simulink model "Senorless"  (R2023a)
settings: Solver=FixedStepDiscrete  StartTime=0.0  StopTime=2  FixedStep=1/FOC_FRQ  RelTol=1e-3
values from neighbouring files (symbols this model uses):
  ADC_REF = 3.6    [Senorless.sldd]
  ADC_SAMPLE_MAX = 32767.0    [Senorless.sldd]
  AMP_GAIN = 32.0    [Senorless.sldd]
  CURR_INPUT = 3276.0    [Senorless.sldd]
  CURR_KI = 380.0    [Senorless.sldd]
  CURR_KP = 0.04    [Senorless.sldd]
  CURR_LIMIT = 1.1    [Senorless.sldd]
  CURR_OVER = 34.0    [Senorless.sldd]
  CURR_POINT_GAIN = 7.0    [Senorless.sldd]
  CURR_STEP = 32760.0    [Senorless.sldd]
  CURR_UNDER = 0.03    [Senorless.sldd]
  CURR_WIDTH = 250.0    [Senorless.sldd]
  FOC_FRQ = 36000.0    [Senorless.sldd]
  GAMMA = 32767.0    [Senorless.sldd]
  HFI_ID = 2.125    [Senorless.sldd]
  IMAX = 34.0    [Senorless.sldd]
  LPF_FRQ = 300.0    [Senorless.sldd]
  MOTOR_DAMPER = 8.3E-7    [Senorless.sldd]
  MOTOR_FLUX = 0.0012713112    [Senorless.sldd]
  MOTOR_INERTIA = 1.02E-6    [Senorless.sldd]
  MOTOR_LS = 1.8E-5    [Senorless.sldd]
  MOTOR_PN = 7.0    [Senorless.sldd]
  MOTOR_RS = 0.065    [Senorless.sldd]
  NS_COMP_UD = 0.531    [Senorless.sldd]
  PLL_LIMIT = 0.95    [Senorless.sldd]
  PLL_WIDTH = 500.0    [Senorless.sldd]
  PWM_FRQ = 96000000.0    [Senorless.sldd]
  RS_HUNT = 0.002    [Senorless.sldd]
  SMOK_FRQ = 1200.0    [Senorless.sldd]
  SPD_LIMIT = 0.8    [Senorless.sldd]
  SPD_LPF_LEVEL = 15.0    [Senorless.sldd]
  SPD_MAX = 8100.0    [Senorless.sldd]
  SPD_MIN = -8100.0    [Senorless.sldd]
  SPD_REDUCE = 380.0    [Senorless.sldd]
  SPD_STEP = 3.0    [Senorless.sldd]
  SPD_WIDTH = 10.0    [Senorless.sldd]
  TS_POINT_GAIN = 10.0    [Senorless.sldd]
  UDC = 17.0    [Senorless.sldd]
  UDC_GAIN = 21.0    [Senorless.sldd]
  UDC_POINT_GAIN = 10.0    [Senorless.sldd]
undefined symbols (not defined in the file or in its folder): curr_q_ki, curr_q_kp, DiscIntNeverNeededParam, magnitude, PLL_LPF_LEVEL, Udc
libraries: simulink x20, slpidlib x5, mcbcontrolslib x4, mcbplantlib x1, autolibpmsminterior x1, autolibpmsmexterior x1, spspowerguiLib x1
(part 4 of 7)

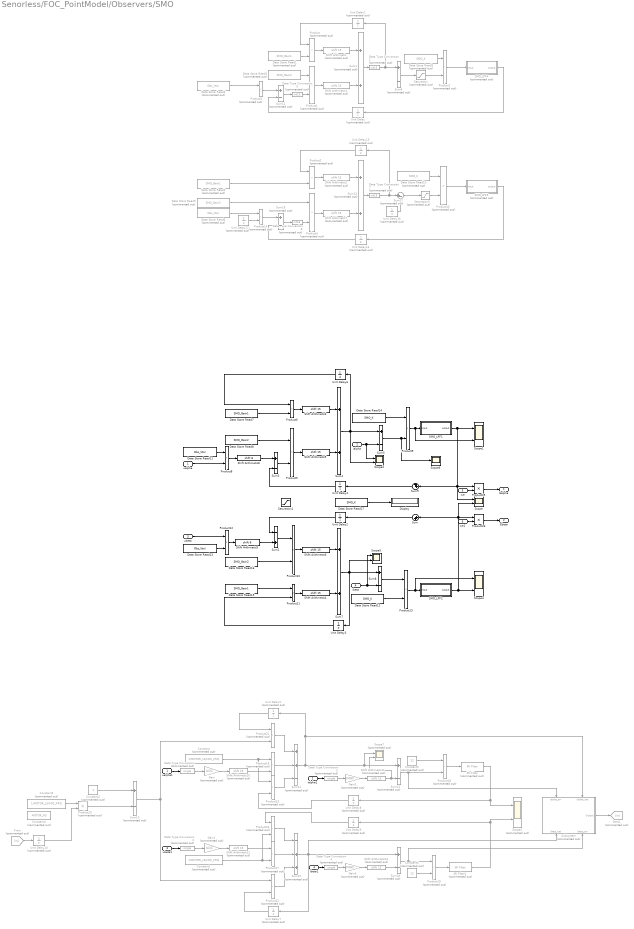
== system Senorless/FOC_PointModel/Observers/SMO ==
  ualpha : Inport
  ialpha : Inport  Port=2
  ubeta : Inport  Port=3
  ibeta : Inport  Port=4
  we : Inport  Port=5
  Constant : Constant  Commented=on  Value=1/MOTOR_LS/FOC_FRQ
  Constant1 : Constant  Commented=on  Value=1/MOTOR_LS/FOC_FRQ
  Constant2 : Constant  Commented=on  OutDataTypeStr=single
  Constant3 : Constant  Commented=on  Value=1/MOTOR_LS/FOC_FRQ
  Constant4 : Constant  Commented=on  Value=MOTOR_RS
  Constant5 : Constant  Commented=on  Value=12  OutDataTypeStr=single
  Constant6 : Constant  Commented=on  Value=12  OutDataTypeStr=single
  Data Store Read1 : DataStoreRead  Commented=on  DataStoreName=SMO_Gain1  IndexOptions=Index vector (dialog)  Indices=1  OutputSizes=1
  Data Store Read10 : DataStoreRead  Commented=on  DataStoreName=SMO_K  IndexOptions=Index vector (dialog)  Indices=1  OutputSizes=1
  Data Store Read11 : DataStoreRead  DataStoreName=Obs_VtoI  IndexOptions=Index vector (dialog)  Indices=1  OutputSizes=1
  Data Store Read12 : DataStoreRead  DataStoreName=SMO_K  IndexOptions=Index vector (dialog)  Indices=1  OutputSizes=1
  Data Store Read13 : DataStoreRead  DataStoreName=Obs_VtoI  IndexOptions=Index vector (dialog)  Indices=1  OutputSizes=1
  Data Store Read14 : DataStoreRead  DataStoreName=SMO_K  IndexOptions=Index vector (dialog)  Indices=1  OutputSizes=1
  Data Store Read15 : DataStoreRead  DataStoreName=SMO_Gain1  IndexOptions=Index vector (dialog)  Indices=1  OutputSizes=1
  Data Store Read16 : DataStoreRead  DataStoreName=SMO_Gain2  IndexOptions=Index vector (dialog)  Indices=1  OutputSizes=1
  Data Store Read17 : DataStoreRead  DataStoreName=SMO_K  IndexOptions=Index vector (dialog)  Indices=1  OutputSizes=1
  Data Store Read2 : DataStoreRead  Commented=on  DataStoreName=SMO_Gain1  IndexOptions=Index vector (dialog)  Indices=1  OutputSizes=1
  Data Store Read3 : DataStoreRead  Commented=on  DataStoreName=SMO_Gain2  IndexOptions=Index vector (dialog)  Indices=1  OutputSizes=1
  Data Store Read4 : DataStoreRead  Commented=on  DataStoreName=Obs_VtoI  IndexOptions=Index vector (dialog)  Indices=1  OutputSizes=1
  Data Store Read5 : DataStoreRead  Commented=on  DataStoreName=SMO_Gain2  IndexOptions=Index vector (dialog)  Indices=1  OutputSizes=1
  Data Store Read6 : DataStoreRead  Commented=on  DataStoreName=Obs_VtoI  IndexOptions=Index vector (dialog)  Indices=1  OutputSizes=1
  Data Store Read7 : DataStoreRead  DataStoreName=SMO_Gain1  IndexOptions=Index vector (dialog)  Indices=1  OutputSizes=1
  Data Store Read8 : DataStoreRead  DataStoreName=SMO_Gain2  IndexOptions=Index vector (dialog)  Indices=1  OutputSizes=1
  Data Store Read9 : DataStoreRead  Commented=on  DataStoreName=SMO_K  IndexOptions=Index vector (dialog)  Indices=1  OutputSizes=1
  Data Type Conversion{,2..4} (4 alike) : DataTypeConversion  Commented=on  OutDataTypeStr=single  SaturateOnIntegerOverflow=off  RndMeth=Floor
  Data Type Conversion{1,5,7..8} (4 alike) : DataTypeConversion  Commented=on  OutDataTypeStr=int16  SaturateOnIntegerOverflow=off
  Display : Display
  From : From  Commented=on  GotoTag=rs
  Gain : Gain  Commented=on  Gain=UDC
  Gain1 : Gain  Commented=on  Gain=UDC
  Gain2 : Gain  Commented=on  Gain=IMAX
  Gain3 : Gain  Commented=on  Gain=IMAX
  Goto1 : Goto  Commented=on  GotoTag=rs
  IIR Filter : mcbcontrolslib/IIR Filter  Commented=on  VariantControl=Low Pass Filter  VariantSelect=Low-pass  Filter_constant=0.07  advancedSettings=off  Ts=50e-6  cutOff_freq=239.5881
      settings: LibrarySourceBlock=mcbhdllib/Signal Management/IIR Filter
  IIR Filter1 : mcbcontrolslib/IIR Filter  Commented=on  VariantControl=Low Pass Filter  VariantSelect=Low-pass  Filter_constant=0.07  advancedSettings=off  Ts=50e-6  cutOff_freq=239.5881
      settings: LibrarySourceBlock=mcbhdllib/Signal Management/IIR Filter
  Product{,1..4,7,14..15} (8 alike) : Product  Commented=on  OutDataTypeStr=int32  RndMeth=Zero
  Product{5..6,8..13,25..26} (10 alike) : Product  OutDataTypeStr=int32  RndMeth=Zero
  Product{16..24} (9 alike) : Product  Commented=on
  SMO_LPF1 : Subsystem
  SMO_LPF2 : Subsystem
  SMO_LPF4 : Subsystem  Commented=on  TreatAsAtomicUnit=on
  SMO_LPF5 : Subsystem  Commented=on  TreatAsAtomicUnit=on
  Saturation : Saturate  Commented=on  UpperLimit=32768*0.5  LowerLimit=-32768*0.5  OutDataTypeStr=int16  RndMeth=Zero
  Saturation1 : Saturate  UpperLimit=32767  LowerLimit=-32767  OutDataTypeStr=int32  RndMeth=Zero
  Saturation3 : Saturate  Commented=on  UpperLimit=32768*0.5  LowerLimit=-32768*0.5  OutDataTypeStr=int16  RndMeth=Zero
  Scope{,1..2,4..5} (5 alike) : Scope  NumInputPorts=2
  Scope3 : Scope  Commented=on  NumInputPorts=2
  Scope6 : Scope
  Scope7 : Scope  Commented=on  NumInputPorts=2
  Shift Arithmetic{,1..2,7,10..13} (8 alike) : ArithShift  Commented=on  BitShiftNumber=15
  Shift Arithmetic{3..6} (4 alike) : ArithShift  BitShiftNumber=15  DiagnosticForOORShift=Error
  Shift Arithmetic8 : ArithShift  BitShiftNumber=8
  Shift Arithmetic9 : ArithShift  BitShiftNumber=8
  Subsystem : Subsystem  Commented=on
      settings: PortSchema="{\"entries\":[{\"content\":{\"sides\":[{\"content\":{},\"type\":\"ConnectorPlacement.EquallySpacedRectSide\",\"uuid\":\"b8d9eb56-9873-4626-b110-f5e82f41559d\"},{\"content\":{\"connectorIds\":[\"Out1\"],\"side\":\"RIGHT\"},\"type\":\"ConnectorPlacement.EquallySpacedRectSide\",\"uuid\":\"658789fc-224b-44e9-b365-546b63f28a3f\"},{\"content\":{\"connectorIds\":[\"In1\",\"In2\"],\"side\":\"TOP\"},\"type\":\"ConnectorPlacement.EquallySpacedRectSide\",\"uuid\":\"05c41f48-0bd2-48b6-962d-dae447ff7d68\"},{\"content\":{\"connectorIds\":[\"In3\",\"In4\"],\"side\":\"BOTTOM\"},\"type\":\"ConnectorPlacement.EquallySpacedRectSide\",\"uuid\":\"829c9f03-f344-43ec-9cb0-3f5e0857c861\"}]},\"type\":\"ConnectorPlacement.EquallySpacedConnector\",\"uuid\":\"ff8d46c8-3816-4d27-98d8-4daa626fea9c\"}],\"packageUris\":[\"http://schema.mathworks.com/mf0/Connector/R2020b\"],\"version\":\"1.0\"}"
  Sum : Sum  Inputs=|++
  Sum1 : Sum  Commented=on
  Sum10 : Sum  Commented=on  Inputs=+-
  Sum11 : Sum  Commented=on  Inputs=++-
  Sum12 : Sum  Commented=on  Inputs=+-
  Sum13 : Sum  Commented=on
  Sum14 : Sum  Commented=on  Inputs=+-  RndMeth=Zero
  Sum15 : Sum  Commented=on  Inputs=-++
  Sum16 : Sum  Commented=on  Inputs=+-
  Sum17 : Sum  Commented=on  Inputs=|+-  OutDataTypeStr=int16  RndMeth=Zero
  Sum18 : Sum  Commented=on  Inputs=+-  RndMeth=Zero
  Sum2 : Sum  Inputs=-+
  Sum3 : Sum  Inputs=+-  OutDataTypeStr=int32  RndMeth=Zero
  Sum4 : Sum  OutDataTypeStr=int32  RndMeth=Zero
  Sum5 : Sum  Inputs=+-  OutDataTypeStr=int32  RndMeth=Zero
  Sum6 : Sum  Commented=on  Inputs=+-  OutDataTypeStr=int16  RndMeth=Zero
  Sum7 : Sum  OutDataTypeStr=int32
  Sum8 : Sum  Inputs=+-  OutDataTypeStr=int32  RndMeth=Zero
  Sum9 : Sum  Inputs=++|
  Unit Delay{,1,5,7..9,14..17} (10 alike) : UnitDelay  Commented=on  SampleTime=-1  HasFrameUpgradeWarning=on
  Unit Delay10 : UnitDelay  Commented=on  InitialCondition=MOTOR_RS  SampleTime=-1  HasFrameUpgradeWarning=on
  Unit Delay{2..4,6} (4 alike) : UnitDelay  SampleTime=-1  HasFrameUpgradeWarning=on
  ialpha1 : InportShadow  Port=2
  ibeta1 : InportShadow  Port=4
  ualpha1 : InportShadow
  ubeta1 : InportShadow  Port=3
  we1 : InportShadow  Port=5
  Ealpha : Outport
  Ebeta : Outport  Port=2
  wires:
  Shift Arithmetic1/1 -> Sum1/2
  Shift Arithmetic2/1 -> Sum13/1
  Data Store Read1/1 -> Product/2
  Data Store Read4/1 -> Product3/1
  Product1/1 -> Shift Arithmetic1/1
  Product3/1 -> Sum12/1
  Unit Delay/1 -> Sum12/2
  Data Type Conversion1/1 -> Sum6/1, Unit Delay1/1
  Sum1/1 -> Data Type Conversion1/1
  Unit Delay1/1 -> Product/1
  Product/1 -> Shift Arithmetic/1
  Saturation3/1 -> Product15/2
  Data Type Conversion7/1 -> Unit Delay15/1, Sum17/1
  Data Store Read5/1 -> Product4/1
  Saturation/1 -> Product7/2
  Product2/1 -> Shift Arithmetic2/1
  Sum12/1 -> Data Type Conversion5/1
  Sum17/1 -> Saturation3/1
  Data Type Conversion5/1 -> Product1/2
  Unit Delay15/1 -> Product2/1
  Shift Arithmetic/1 -> Sum1/1
  Unit Delay14/1 -> Sum16/2
  Sum13/1 -> Data Type Conversion7/1
  Data Type Conversion8/1 -> Product4/2
  Data Store Read2/1 -> Product2/2
  Shift Arithmetic7/1 -> Sum13/2
  Product4/1 -> Shift Arithmetic7/1
  Unit Delay17/1 -> Product14/2
  Product14/1 -> Sum16/1
  Sum16/1 -> Data Type Conversion8/1
  Data Store Read6/1 -> Product14/1
  Unit Delay16/1 -> Sum17/2
  Data Store Read3/1 -> Product1/1
  Data Store Read9/1 -> Product7/1
  Data Store Read10/1 -> Product15/1
  Product15/1 -> SMO_LPF5/1(input)
  Product7/1 -> SMO_LPF4/1(input)
  SMO_LPF4/1(output) -> Unit Delay/1
  SMO_LPF5/1(output) -> Unit Delay14/1
  Data Store Read8/1 -> Product5/1
  Product6/1 -> Shift Arithmetic3/1
  Product5/1 -> Shift Arithmetic5/1
  Sum6/1 -> Saturation/1
  Product10/1 -> Shift Arithmetic6/1
  Product11/1 -> Shift Arithmetic4/1
  Shift Arithmetic3/1 -> Sum4/1
  Shift Arithmetic5/1 -> Sum4/2
  Data Store Read17/1 -> Display/1
  Data Store Read14/1 -> Product9/1
  Sum7/1 -> Scope5/2, Unit Delay3/1, Sum8/1
  Sum4/1 -> Sum5/1, Scope2/2, Unit Delay6/1
  Sum/1 -> Unit Delay2/1
  Sum9/1 -> Unit Delay4/1
  ialpha/1 -> Scope2/1, Sum5/2
  ibeta/1 -> Scope5/1, Sum8/2
  Unit Delay6/1 -> Product6/1
  Product13/1 -> SMO_LPF2/1(input), Scope4/1
  Shift Arithmetic6/1 -> Sum7/1
  Data Store Read16/1 -> Product10/2
  Shift Arithmetic4/1 -> Sum7/2
  Unit Delay3/1 -> Product11/2
  Data Store Read12/1 -> Product13/2
  Subsystem/1(Output) -> Goto1/1
  Data Store Read7/1 -> Product6/2
  Data Store Read15/1 -> Product11/1
  Sum8/1 -> Product13/1
  Sum3/1 -> Product5/2
  Product8/1 -> Shift Arithmetic8/1
  Data Store Read11/1 -> Product8/1
  Unit Delay4/1 -> Sum3/2
  Sum2/1 -> Product10/1
  Shift Arithmetic9/1 -> Sum2/2
  Product12/1 -> Shift Arithmetic9/1
  Data Store Read13/1 -> Product12/2
  Unit Delay2/1 -> Sum2/1
  SMO_LPF2/1(output) -> Scope4/2, Product26/1, Sum/1, Scope/2
  Sum5/1 -> Scope6/1, Product9/2
  ualpha1/1 -> Data Type Conversion/1
  ubeta1/1 -> Data Type Conversion2/1
  ialpha1/1 -> Data Type Conversion3/1
  ibeta1/1 -> Data Type Conversion4/1
  Gain/1 -> Shift Arithmetic10/1
  Gain1/1 -> Shift Arithmetic12/1
  Gain3/1 -> Shift Arithmetic13/1
  Gain2/1 -> Shift Arithmetic11/1
  Shift Arithmetic10/1 -> Product16/2
  Constant/1 -> Product23/1, Product16/1
  Constant1/1 -> Product24/2, Product17/2
  Constant2/1 -> Sum10/1
  Product20/1 -> Sum10/2
  Constant3/1 -> Product20/1
  Sum10/1 -> Product22/1, Product21/2
  Product16/1 -> Sum11/2
  Product21/1 -> Sum11/1
  Sum11/1 -> Scope7/1, Sum14/1, Subsystem/2(ialpha_hat), Unit Delay5/1
  Unit Delay5/1 -> Product21/1
  Shift Arithmetic11/1 -> Scope7/2, Sum14/2
  Constant5/1 -> Product18/1
  Product18/1 -> IIR Filter/1
  IIR Filter/1 -> Scope3/1, Unit Delay8/1
  Sum15/1 -> Subsystem/3(ibeta_hat), Unit Delay7/1, Sum18/1
  Shift Arithmetic13/1 -> Sum18/2
  Product17/1 -> Sum15/2
  Product22/1 -> Sum15/3
  Constant6/1 -> Product19/2
  Product19/1 -> IIR Filter1/1
  IIR Filter1/1 -> Scope3/2, Unit Delay9/1
  Unit Delay7/1 -> Product22/2
  Data Type Conversion/1 -> Gain/1
  Data Type Conversion2/1 -> Gain1/1
  Data Type Conversion3/1 -> Gain2/1
  Data Type Conversion4/1 -> Gain3/1
  Unit Delay8/1 -> Product23/2
  SMO_LPF1/1(output) -> Product25/1, Sum9/2, Scope/1, Scope1/1
  ubeta/1 -> Product12/1
  ualpha/1 -> Product8/2
  Product9/1 -> Scope1/2, SMO_LPF1/1(input)
  Shift Arithmetic8/1 -> Sum3/1
  Shift Arithmetic12/1 -> Product17/1
  Unit Delay9/1 -> Product24/1
  Product24/1 -> Sum15/1
  Product23/1 -> Sum11/3
  From/1 -> Unit Delay10/1
  Sum14/1 -> Product18/2, Subsystem/1(ialpha_err)
  Sum18/1 -> Product19/1, Subsystem/4(ibeta_err)
  Unit Delay10/1 -> Product20/2
  we/1 -> Product25/2
  Product25/1 -> Ealpha/1
  Product26/1 -> Ebeta/1
  we1/1 -> Product26/2

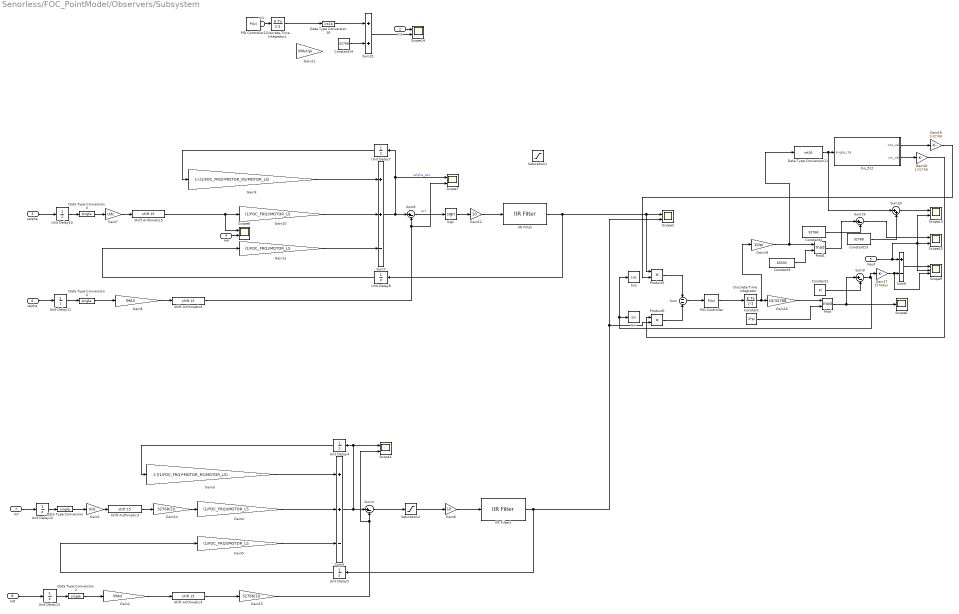
== system Senorless/FOC_PointModel/Observers/Subsystem ==
  In1 : Inport
  In2 : Inport  Port=2
  ualpha : Inport  Port=3
  In4 : Inport  Port=4
  Input : Inport  Port=5
  ialpha : Inport  Port=6
  In7 : Inport  Port=7
  In8 : Inport  Port=8
  Constant : Constant  Value=2*pi  OutDataTypeStr=single
  Constant1 : Constant  Value=pi  OutDataTypeStr=single
  Constant13 : Constant  Value=32768  OutDataTypeStr=int16
  Constant14 : Constant  Value=32768  OutDataTypeStr=int16
  Constant3 : Constant  Value=65535  OutDataTypeStr=single
  Constant4 : Constant  Value=32768
  Cos : Trigonometry  Operator=cos
  Data Type Conversion{,2..4} (4 alike) : DataTypeConversion  OutDataTypeStr=single  SaturateOnIntegerOverflow=off  RndMeth=Floor
  Data Type Conversion11 : DataTypeConversion  OutDataTypeStr=int16  SaturateOnIntegerOverflow=off  RndMeth=Floor
  Data Type Conversion16 : DataTypeConversion  OutDataTypeStr=int16  SaturateOnIntegerOverflow=off
  Discrete-Time Integrator : DiscreteIntegrator  SampleTime=-1  ICPrevOutput=DiscIntNeverNeededParam  ICPrevScaledInput=DiscIntNeverNeededParam
  Discrete-Time Integrator1 : DiscreteIntegrator  SampleTime=-1  OutDataTypeStr=int32  RndMeth=Zero  ICPrevOutput=DiscIntNeverNeededParam  ICPrevScaledInput=DiscIntNeverNeededParam
  Gain1 : Gain  Gain=Udc
  Gain10 : Gain  Gain=(1/FOC_FRQ)/MOTOR_LS
  Gain11 : Gain  Gain=(1/FOC_FRQ)/MOTOR_LS  OutDataTypeStr=single
  Gain12 : Gain  Gain=10
  Gain14 : Gain  Gain=32768/10
  Gain15 : Gain  Gain=32768/10
  Gain16 : Gain  Gain=10/32768
  Gain17 : Gain  Gain=32768/pi
  Gain18 : Gain  Gain=10/pi
  Gain19 : Gain  Gain=1/32768  OutDataTypeStr=single
  Gain2 : Gain  Gain=IMAX
  Gain20 : Gain  Gain=1/32768  OutDataTypeStr=single
  Gain21 : Gain  Gain=IMAX/pi  OutDataTypeStr=int32  RndMeth=Zero
  Gain3 : Gain  Gain=1-((1/FOC_FRQ)*MOTOR_RS/MOTOR_LS)  OutDataTypeStr=single
  Gain4 : Gain  Gain=(1/FOC_FRQ)/MOTOR_LS
  Gain5 : Gain  Gain=(1/FOC_FRQ)/MOTOR_LS  OutDataTypeStr=single
  Gain6 : Gain  Gain=10
  Gain7 : Gain  Gain=Udc
  Gain8 : Gain  Gain=IMAX
  Gain9 : Gain  Gain=1-((1/FOC_FRQ)*MOTOR_RS/MOTOR_LS)  OutDataTypeStr=single
  IIR Filter : mcbcontrolslib/IIR Filter  VariantControl=Low Pass Filter  VariantSelect=Low-pass  Filter_constant=0.1  advancedSettings=off  Ts=50e-6  cutOff_freq=353.6777
      settings: LibrarySourceBlock=mcbhdllib/Signal Management/IIR Filter
  IIR Filter1 : mcbcontrolslib/IIR Filter  VariantControl=Low Pass Filter  VariantSelect=Low-pass  Filter_constant=0.149  advancedSettings=off  Ts=50e-6  cutOff_freq=557.3228
      settings: LibrarySourceBlock=mcbhdllib/Signal Management/IIR Filter
  Mod : Math  Operator=mod
  Mod1 : Math  Operator=mod
  PID Controller : slpidlib/PID Controller  Controller=PI  Form=Parallel  TimeDomain=Discrete-time  UseExternalTs=off  SampleTime=-1  IntegratorMethod=Forward Euler  FilterMethod=Forward Euler  ControllerParametersSource=internal  P=2*0.707*100  I=100*100  UseKiTs=off  D=0  N=100  UseFilter=on  TunerSelectOption=Transfer Function Based (PID Tuner App)  InitialConditionSource=internal  InitialConditionForIntegrator=0  InitialConditionForFilter=0  DifferentiatorICPrevScaledInput=0  ExternalReset=none  TrackingMode=off  Kt=1  LimitOutput=off  SatLimitsSource=internal  UpperSaturationLimit=inf  LowerSaturationLimit=-inf  LinearizeAsGain=on  AntiWindupMode=none  Kb=1  LimitIntegrator=off  UpperIntegratorSaturationLimit=inf  LowerIntegratorSaturationLimit=-inf  POutMin=[]  POutMax=[]  IOutMin=[]  IOutMax=[]  DOutMin=[]  DOutMax=[]  NOutMin=[]  NOutMax=[]  SumOutMin=[]  SumOutMax=[]  SaturationOutMin=[]  SaturationOutMax=[]  PParamMin=[]  PParamMax=[]  IParamMin=[]  IParamMax=[]  DParamMin=[]  DParamMax=[]  NParamMin=[]  NParamMax=[]  KbParamMin=[]  KbParamMax=[]  KtParamMin=[]  KtParamMax=[]  KbOutMin=[]  KbOutMax=[]  KtOutMin=[]  KtOutMax=[]  IntegratorOutMin=[]  IntegratorOutMax=[]  FilterOutMin=[]  FilterOutMax=[]  SumI1OutMin=[]  SumI1OutMax=[]  SumI2OutMin=[]  SumI2OutMax=[]  SumI3OutMin=[]  SumI3OutMax=[]  SumI4OutMin=[]  SumI4OutMax=[]  SumDOutMin=[]  SumDOutMax=[]  DifferentiatorOutMin=[]  DifferentiatorOutMax=[]  FilterDiffOutCoefMin=[]  FilterDiffOutCoefMax=[]  ReciprocalOutMin=[]  ReciprocalOutMax=[]  SumDenOutMin=[]  SumDenOutMax=[]  SumNumOutMin=[]  SumNumOutMax=[]  DivideOutMin=[]  DivideOutMax=[]  UdiffTsProdOutMin=[]  UdiffTsProdOutMax=[]  NTsProdOutMin=[]  NTsProdOutMax=[]  UintegralTsProdOutMin=[]  UintegralTsProdOutMax=[]  UngainTsProdOutMin=[]  UngainTsProdOutMax=[]  ClampingZeroOutDataTypeStr=Inherit: Inherit via back propagation  ClampingZeroOutMin=[]  ClampingZeroOutMax=[]  FilterDenConstantOutDataTypeStr=Inherit: Inherit via back propagation  FilterDenConstantOutMin=[]  FilterDenConstantOutMax=[]  PCopyOutDataTypeStr=Inherit: Inherit via back propagation  PCopyOutMin=[]  PCopyOutMax=[]  NCopyOutDataTypeStr=Inherit: Inherit via back propagation  NCopyOutMin=[]  NCopyOutMax=[]  IntegratorContinuousStateAttributes=''  IntegratorStateMustResolveToSignalObject=off  IntegratorRTWStateStorageClass=Auto  FilterContinuousStateAttributes=''  FilterStateMustResolveToSignalObject=off  FilterRTWStateStorageClass=Auto  ParallelPVariant=InternalParameters  IdealPVariant=Disabled  IVariant=InternalParameters  DVariant=Disabled  IntegratorVariant=Discrete  SatVariant=Disabled  AWVariant=Passthrough  PCopyVariant=Disabled  TRVariant=Disabled  FdbkBlocksVariant=Forward  IdealPFdbkVariant=Disabled  SatFdbkVariant=Disabled  DerivativeFilterVariant=Disabled  NVariant=Disabled  NCopyVariant=Disabled_SignalSpec  FilterICVariant=Disabled  IntegratorICVariant=InternalICs  ExternalResetVariant=Disabled  TRSumVariant=Passthrough  SumFdbkVariant=Disabled  SumVariant=Sum_PI  TsampFilterVariant=InternalTs  TsampNgainVariant=Passthrough  TsampIntegralVariant=Disabled_SignalSpec  ExternalSaturationOutDataTypeStr=Inherit: Same as second input
  PID Controller1 : slpidlib/PID Controller  Controller=PI  Form=Parallel  TimeDomain=Discrete-time  UseExternalTs=off  SampleTime=-1  IntegratorMethod=Forward Euler  FilterMethod=Forward Euler  ControllerParametersSource=internal  P=2*0.707*100  I=100*100  UseKiTs=off  D=0  N=100  UseFilter=on  TunerSelectOption=Transfer Function Based (PID Tuner App)  InitialConditionSource=internal  InitialConditionForIntegrator=0  InitialConditionForFilter=0  DifferentiatorICPrevScaledInput=0  ExternalReset=none  TrackingMode=off  Kt=1  LimitOutput=off  SatLimitsSource=internal  UpperSaturationLimit=inf  LowerSaturationLimit=-inf  LinearizeAsGain=on  AntiWindupMode=none  Kb=1  LimitIntegrator=off  UpperIntegratorSaturationLimit=inf  LowerIntegratorSaturationLimit=-inf  PGainOutDataTypeStr=int32  PProdOutDataTypeStr=int32  POutMin=[]  POutMax=[]  IGainOutDataTypeStr=int32  IProdOutDataTypeStr=int32  IOutMin=[]  IOutMax=[]  DOutMin=[]  DOutMax=[]  NOutMin=[]  NOutMax=[]  SumOutDataTypeStr=int32  SumOutMin=[]  SumOutMax=[]  SaturationOutMin=[]  SaturationOutMax=[]  PParamDataTypeStr=int16  PParamMin=[]  PParamMax=[]  IParamDataTypeStr=int16  IParamMin=[]  IParamMax=[]  DParamMin=[]  DParamMax=[]  NParamMin=[]  NParamMax=[]  KbParamMin=[]  KbParamMax=[]  KtParamMin=[]  KtParamMax=[]  KbOutMin=[]  KbOutMax=[]  KtOutMin=[]  KtOutMax=[]  IntegratorOutDataTypeStr=int32  IntegratorOutMin=[]  IntegratorOutMax=[]  FilterOutMin=[]  FilterOutMax=[]  SumI1OutMin=[]  SumI1OutMax=[]  SumI2OutMin=[]  SumI2OutMax=[]  SumI3OutMin=[]  SumI3OutMax=[]  SumI4OutMin=[]  SumI4OutMax=[]  SumDOutMin=[]  SumDOutMax=[]  SumAccumDataTypeStr=int32  DifferentiatorOutMin=[]  DifferentiatorOutMax=[]  FilterDiffOutCoefMin=[]  FilterDiffOutCoefMax=[]  ReciprocalOutMin=[]  ReciprocalOutMax=[]  SumDenOutMin=[]  SumDenOutMax=[]  SumNumOutMin=[]  SumNumOutMax=[]  DivideOutMin=[]  DivideOutMax=[]  UdiffTsProdOutMin=[]  UdiffTsProdOutMax=[]  NTsProdOutMin=[]  NTsProdOutMax=[]  UintegralTsProdOutMin=[]  UintegralTsProdOutMax=[]  UngainTsProdOutMin=[]  UngainTsProdOutMax=[]  ClampingZeroOutDataTypeStr=Inherit: Inherit via back propagation  ClampingZeroOutMin=[]  ClampingZeroOutMax=[]  FilterDenConstantOutDataTypeStr=Inherit: Inherit via back propagation  FilterDenConstantOutMin=[]  FilterDenConstantOutMax=[]  PCopyOutDataTypeStr=Inherit: Inherit via back propagation  PCopyOutMin=[]  PCopyOutMax=[]  NCopyOutDataTypeStr=Inherit: Inherit via back propagation  NCopyOutMin=[]  NCopyOutMax=[]  IntegratorContinuousStateAttributes=''  IntegratorStateMustResolveToSignalObject=off  IntegratorRTWStateStorageClass=Auto  FilterContinuousStateAttributes=''  FilterStateMustResolveToSignalObject=off  FilterRTWStateStorageClass=Auto  ParallelPVariant=InternalParameters  IdealPVariant=Disabled  IVariant=InternalParameters  DVariant=Disabled  IntegratorVariant=Discrete  SatVariant=Disabled  AWVariant=Passthrough  PCopyVariant=Disabled  TRVariant=Disabled  FdbkBlocksVariant=Forward  IdealPFdbkVariant=Disabled  SatFdbkVariant=Disabled  DerivativeFilterVariant=Disabled  NVariant=Disabled  NCopyVariant=Disabled_SignalSpec  FilterICVariant=Disabled  IntegratorICVariant=InternalICs  ExternalResetVariant=Disabled  TRSumVariant=Passthrough  SumFdbkVariant=Disabled  SumVariant=Sum_PI  TsampFilterVariant=InternalTs  TsampNgainVariant=Passthrough  TsampIntegralVariant=Disabled_SignalSpec  ExternalSaturationOutDataTypeStr=Inherit: Same as second input
  Product5 : Product
  Product6 : Product
  Saturation1 : Saturate  UpperLimit=32768  LowerLimit=-32768
  Saturation2 : Saturate  UpperLimit=32768  LowerLimit=-32768
  Scope{2..3,7..8,10,13..14} (7 alike) : Scope  NumInputPorts=2
  Scope6 : Scope
  Scope9 : Scope  NumInputPorts=3
  Shift Arithmetic{3..6} (4 alike) : ArithShift  BitShiftNumber=15
  Sign : Signum
  Sin : Trigonometry
  Sin_512 : MATLAB Function  TreatAsAtomicUnit=on
  Sum : Sum  Inputs=--
  Sum19 : Sum  Inputs=|+-
  Sum20 : Sum  Inputs=|++
  Sum21 : Sum
  Sum3 : Sum  Inputs=++-
  Sum4 : Sum  Inputs=|+-  RndMeth=Zero
  Sum6 : Sum  Inputs=+-
  Sum7 : Sum  Inputs=++-
  Sum8 : Sum  Inputs=|+-  RndMeth=Zero
  Sum9 : Sum  Inputs=|+-
  Unit Delay{4..5,7..8,10..13} (8 alike) : UnitDelay  SampleTime=-1  HasFrameUpgradeWarning=on
  wires:
  Sum8/1 -> Sign/1  "err"
  Gain3/1 -> Sum3/1
  Sum9/1 -> Cos/1, Sin/1, Gain17/1
  Saturation2/1 -> Gain6/1
  Unit Delay11/1 -> Data Type Conversion4/1
  Sum7/1 -> Unit Delay7/1, Scope7/1, Sum8/1  "ialpha_est"
  IIR Filter1/1 -> Unit Delay5/1, Scope2/2, Product6/2
  Data Type Conversion4/1 -> Gain8/1
  Unit Delay10/1 -> Data Type Conversion3/1
  Gain18/1 -> Mod1/1, Data Type Conversion11/1
  Gain20/1 -> Product6/1
  Sin_512/1(cos_val) -> Gain19/1
  Product5/1 -> Sum/1
  Gain15/1 -> Scope3/2, Sum4/2
  Sum4/1 -> Saturation2/1
  Input/1 -> Scope13/2, Scope9/2, Scope10/2, Sum6/1
  Gain4/1 -> Sum3/2
  Shift Arithmetic3/1 -> Gain14/1
  Gain2/1 -> Shift Arithmetic4/1
  Shift Arithmetic5/1 -> Scope8/1, Gain10/1
  Sum3/1 -> Scope3/1, Unit Delay4/1, Sum4/1
  Data Type Conversion3/1 -> Gain7/1
  Constant14/1 -> Sum21/2
  Unit Delay4/1 -> Gain3/1
  Gain1/1 -> Shift Arithmetic3/1
  Gain10/1 -> Sum7/2
  Discrete-Time Integrator1/1 -> Data Type Conversion16/1
  Sum21/1 -> Scope14/2
  Shift Arithmetic6/1 -> Scope7/2, Sum8/2
  Data Type Conversion/1 -> Gain1/1
  Shift Arithmetic4/1 -> Gain15/1
  Sign/1 -> Gain12/1
  Constant3/1 -> Mod1/2
  Gain8/1 -> Shift Arithmetic6/1
  Gain11/1 -> Sum7/3
  Unit Delay12/1 -> Data Type Conversion/1
  ialpha/1 -> Unit Delay11/1
  Unit Delay7/1 -> Gain9/1
  Unit Delay13/1 -> Data Type Conversion2/1
  Data Type Conversion2/1 -> Gain2/1
  Sum19/1 -> Scope10/1
  Gain5/1 -> Sum3/3
  Gain7/1 -> Shift Arithmetic5/1
  Constant/1 -> Mod/2
  Unit Delay5/1 -> Gain5/1
  ualpha/1 -> Unit Delay10/1
  Unit Delay8/1 -> Gain11/1
  Gain9/1 -> Sum7/1
  Mod/1 -> Sum9/1, Scope6/1
  Discrete-Time Integrator/1 -> Gain18/1, Gain16/1
  Gain17/1 -> Scope9/3, Sum6/2
  Constant4/1 -> Sum19/2
  IIR Filter/1 -> Unit Delay8/1, Product5/1, Scope2/1
  PID Controller/1 -> Discrete-Time Integrator/1
  Gain16/1 -> Mod/1
  Data Type Conversion16/1 -> Sum21/1
  Sin_512/2(sin_val) -> Gain20/1
  Constant1/1 -> Sum9/2
  Mod1/1 -> Sum19/1
  Gain19/1 -> Product5/2
  Constant13/1 -> Sum20/2
  Sum6/1 -> Scope9/1
  Gain6/1 -> IIR Filter1/1
  Data Type Conversion11/1 -> Sum20/1, Sin_512/1(angle_i16)
  Gain12/1 -> IIR Filter/1
  Sum20/1 -> Scope13/1
  Gain14/1 -> Gain4/1
  In2/1 -> Scope14/1
  Product6/1 -> Sum/2
  Sum/1 -> PID Controller/1
  In4/1 -> Scope8/2
  In7/1 -> Unit Delay12/1
  In8/1 -> Unit Delay13/1
  In1/1 -> Discrete-Time Integrator1/1

== system Senorless/FOC_PointModel/Observers/提取波 ==
  In1 : Inport
  In2 : Inport  Port=2
  In3 : Inport  Port=3
  In4 : Inport  Port=4
  Delay4 : Delay  DelayLength=1
  Demux : Demux
  Mux : Mux
  Shift Arithmetic4 : ArithShift  BitShiftNumber=1
  Sum4 : Sum  Inputs=|++
  Out1 : Outport
  Out2 : Outport  Port=2
  Out3 : Outport  Port=3
  Out4 : Outport  Port=4
  wires:
  Demux/1 -> Out1/1
  In1/1 -> Mux/1
  In2/1 -> Mux/2
  In3/1 -> Mux/3
  In4/1 -> Mux/4
  Sum4/1 -> Shift Arithmetic4/1
  Delay4/1 -> Sum4/2
  Mux/1 -> Delay4/1, Sum4/1
  Shift Arithmetic4/1 -> Demux/1
  Demux/2 -> Out2/1
  Demux/3 -> Out3/1
  Demux/4 -> Out4/1

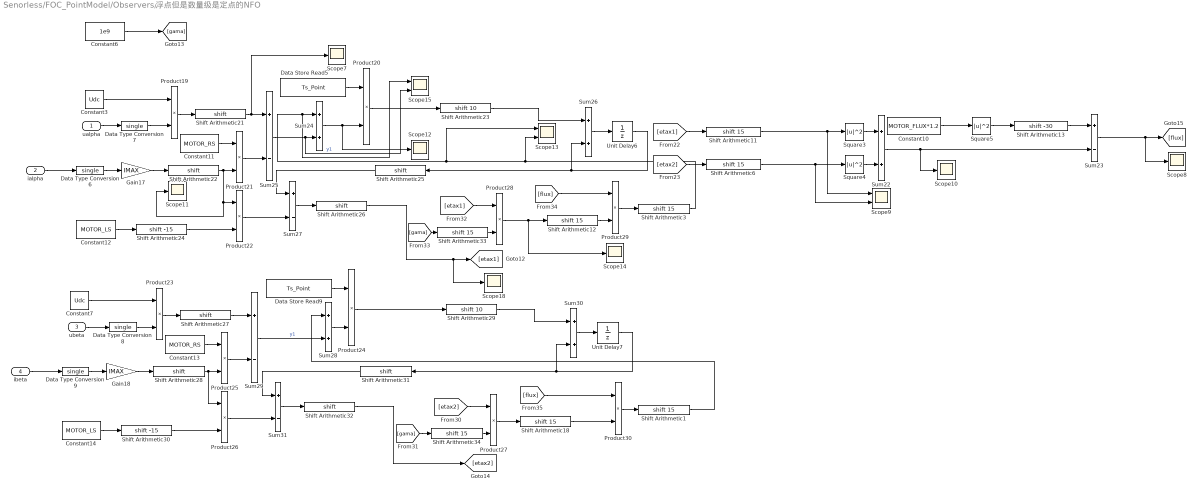
== system Senorless/FOC_PointModel/Observers/浮点但是数量级是定点的NFO ==
  ualpha : Inport
  ialpha : Inport  Port=2
  ubeta : Inport  Port=3
  ibeta : Inport  Port=4
  Constant10 : Constant  Value=MOTOR_FLUX*1.2  OutDataTypeStr=single
  Constant11 : Constant  Value=MOTOR_RS  OutDataTypeStr=single
  Constant12 : Constant  Value=MOTOR_LS  OutDataTypeStr=single
  Constant13 : Constant  Value=MOTOR_RS  OutDataTypeStr=single
  Constant14 : Constant  Value=MOTOR_LS  OutDataTypeStr=single
  Constant3 : Constant  Value=Udc  OutDataTypeStr=single
  Constant6 : Constant  Value=1e9  OutDataTypeStr=uint32
  Constant7 : Constant  Value=Udc  OutDataTypeStr=single
  Data Store Read5 : DataStoreRead  DataStoreName=Ts_Point  IndexOptions=Index vector (dialog)  Indices=1  OutputSizes=1
  Data Store Read9 : DataStoreRead  DataStoreName=Ts_Point  IndexOptions=Index vector (dialog)  Indices=1  OutputSizes=1
  Data Type Conversion{6..9} (4 alike) : DataTypeConversion  OutDataTypeStr=single  SaturateOnIntegerOverflow=off  RndMeth=Floor
  Gain17 : Gain  Gain=IMAX  ParamDataTypeStr=single  OutDataTypeStr=single  RndMeth=Zero
  Gain18 : Gain  Gain=IMAX  ParamDataTypeStr=int16  OutDataTypeStr=single  RndMeth=Zero
  Product{19..30} (12 alike) : Product  OutDataTypeStr=single  RndMeth=Zero
  Scope{7..8,10..12,14,18} (7 alike) : Scope
  Scope13 : Scope  NumInputPorts=2
  Scope15 : Scope  NumInputPorts=2
  Scope9 : Scope  NumInputPorts=2
  Shift Arithmetic{1,3,6,11..12,18,33..34} (8 alike) : ArithShift  BitShiftNumber=15
  Shift Arithmetic13 : ArithShift  BitShiftNumber=-30
  Shift Arithmetic{21..22,25..28,31..32} (8 alike) : ArithShift
  Shift Arithmetic23 : ArithShift  BitShiftNumber=10
  Shift Arithmetic24 : ArithShift  BitShiftNumber=-15
  Shift Arithmetic29 : ArithShift  BitShiftNumber=10
  Shift Arithmetic30 : ArithShift  BitShiftNumber=-15
  Square3 : Math  Operator=magnitude^2
  Square4 : Math  Operator=magnitude^2
  Square5 : Math  Operator=magnitude^2
  Sum{22,24,26,28,30} (5 alike) : Sum  OutDataTypeStr=single  RndMeth=Zero
  Sum{23,25,27,29,31} (5 alike) : Sum  Inputs=+-  OutDataTypeStr=single  RndMeth=Zero
  Unit Delay6 : UnitDelay  SampleTime=-1  HasFrameUpgradeWarning=on
  Unit Delay7 : UnitDelay  SampleTime=-1  HasFrameUpgradeWarning=on
  wires:
  Product25/1 -> Sum29/2
  Shift Arithmetic29/1 -> Sum30/1
  Product24/1 -> Shift Arithmetic29/1
  Product26/1 -> Sum31/2
  Unit Delay6/1 -> Sum26/2, Shift Arithmetic25/1
  Gain17/1 -> Shift Arithmetic22/1
  Shift Arithmetic11/1 -> Scope9/1, Square3/1
  Constant7/1 -> Product23/1
  Shift Arithmetic13/1 -> Sum23/1
  Gain18/1 -> Shift Arithmetic28/1
  Sum31/1 -> Shift Arithmetic32/1
  Shift Arithmetic3/1 -> Scope13/1, Scope15/1, Sum24/1, Scope13/2
  Shift Arithmetic28/1 -> Product26/1, Product25/2
  Unit Delay7/1 -> Sum30/2, Shift Arithmetic31/1
  Sum22/1 -> Scope10/1, Sum23/2
  Sum29/1 -> Sum28/2  "y1"
  Data Type Conversion6/1 -> Gain17/1
  Shift Arithmetic27/1 -> Sum29/1
  [flux] -> Product30/1
  Data Type Conversion8/1 -> Product23/2
  Shift Arithmetic23/1 -> Sum26/1
  Constant13/1 -> Product25/1
  Sum23/1 -> Scope8/1, [flux]
  Product27/1 -> Shift Arithmetic18/1
  Data Store Read9/1 -> Product24/1
  Sum28/1 -> Product24/2
  Sum24/1 -> Scope12/1, Product20/2
  Constant14/1 -> Shift Arithmetic30/1
  Sum30/1 -> Unit Delay7/1
  Shift Arithmetic25/1 -> Sum27/1
  Constant12/1 -> Shift Arithmetic24/1
  Shift Arithmetic31/1 -> Sum31/1
  Constant3/1 -> Product19/1
  Product23/1 -> Shift Arithmetic27/1
  Shift Arithmetic6/1 -> Scope9/2, Square4/1
  Shift Arithmetic34/1 -> Product27/2
  Square5/1 -> Shift Arithmetic13/1
  Square3/1 -> Sum22/1
  Product19/1 -> Shift Arithmetic21/1
  Sum26/1 -> Unit Delay6/1
  [etax1] -> Product28/1
  Sum27/1 -> Shift Arithmetic26/1
  Product29/1 -> Shift Arithmetic3/1
  Shift Arithmetic12/1 -> Product29/2
  ibeta/1 -> Data Type Conversion9/1
  [flux] -> Product29/1
  Constant11/1 -> Product21/1
  Product28/1 -> Scope14/1, Shift Arithmetic12/1
  Product22/1 -> Sum27/2
  Shift Arithmetic32/1 -> [etax2]
  Product21/1 -> Sum25/2
  Shift Arithmetic22/1 -> Product22/1, Scope11/1, Product21/2
  Shift Arithmetic33/1 -> Product28/2
  Sum25/1 -> Scope15/2, Sum24/2  "y1"
  [gama] -> Shift Arithmetic34/1
  Square4/1 -> Sum22/2
  Product20/1 -> Shift Arithmetic23/1
  ualpha/1 -> Data Type Conversion7/1
  [gama] -> Shift Arithmetic33/1
  Constant10/1 -> Square5/1
  Shift Arithmetic18/1 -> Product30/2
  Shift Arithmetic26/1 -> Scope18/1, [etax1]
  [etax2] -> Product27/1
  [etax1] -> Shift Arithmetic11/1
  Data Type Conversion9/1 -> Gain18/1
  ialpha/1 -> Data Type Conversion6/1
  Shift Arithmetic21/1 -> Scope7/1, Sum25/1
  Shift Arithmetic30/1 -> Product26/2
  Product30/1 -> Shift Arithmetic1/1
  Shift Arithmetic24/1 -> Product22/2
  [etax2] -> Shift Arithmetic6/1
  Shift Arithmetic1/1 -> Sum28/1
  Data Type Conversion7/1 -> Product19/2
  ubeta/1 -> Data Type Conversion8/1
  Data Store Read5/1 -> Product20/1
  Constant6/1 -> [gama]

== system Senorless/FOC_PointModel/Observers/滤波器 ==
  input : Inport
  Constant13 : Constant  Value=2*pi*150  OutDataTypeStr=int32
  LPF : Subsystem  TreatAsAtomicUnit=on
  Product : Product  OutDataTypeStr=int32  RndMeth=Zero
  Product1 : Product  OutDataTypeStr=int32  RndMeth=Zero
  Scope : Scope  NumInputPorts=2
  Sum5 : Sum  Inputs=-+|  AccumDataTypeStr=int32  OutDataTypeStr=int32  RndMeth=Zero
  Sum8 : Sum  Inputs=|+-  AccumDataTypeStr=int32  OutDataTypeStr=int32  RndMeth=Zero
  Unit Delay : UnitDelay  SampleTime=-1  HasFrameUpgradeWarning=on
  input1 : InportShadow
  积分器4 : Subsystem
      settings: MinAlgLoopOccurrences=on
  积分器5 : Subsystem
      settings: MinAlgLoopOccurrences=on
  output : Outport
  wires:
  Constant13/1 -> Product/2, Product1/1
  Product/1 -> 积分器4/1(input)
  Product1/1 -> 积分器5/1(input)
  Sum8/1 -> Product/1
  input1/1 -> Scope/2
  积分器4/1(output) -> Unit Delay/1
  Unit Delay/1 -> Sum5/1, Product1/2
  积分器5/1(output) -> LPF/1(input), Sum8/2
  input/1 -> Sum5/2
  Sum5/1 -> Sum8/1
  LPF/1(output) -> output/1, Scope/1
